simulink model "Vector_Control_SVPWM_encoderless_learn_v1_0"  (Simulink 10.0)
settings: Solver=ode23tb  StartTime=0.0  StopTime=2  FixedStep=Ts  RelTol=1e-3
PreLoadFcn:
  | %MotorParamInit_IM.m;
InitFcn:
  | Ts=1e-6;
  | %resolute=100;
  | 
  | run('MotorParamInit_IM.m');
undefined symbols (not defined in the file or in its folder): fN, J, Llr, Lls, np, PN, Rr, Rs, VN
libraries: powerlib x15, sfundemos x2, simulink x2, powerlib_extras x1
Description:
  | Copyright 2011-2013 Ruan Jiayang, Tsinghua Univ.
settings Model: Creator=Hoang Lehuy, Laval University  LastModifiedBy=W002220B  ExtModeTrigMode=oneshot  ExtModeArmWhenConnect=off  ExtModeAutoUpdateStatusClock=off
settings SolverCC: ZeroCrossControl=DisableAll
settings DataIOCC: SaveFinalState=on  SignalLoggingSaveFormat=ModelDataLogs  SaveOutput=off  SaveTime=off  SignalLoggingName=sigsOut
settings OptimizationCC: BlockReduction=off  ExpressionDepthLimit=2147483647  InitFltsAndDblsToZero=on
settings DebuggingCC: SaveWithParameterizedLinksMsg=none  CheckExecutionContextPreStartOutputMsg=on  CheckExecutionContextRuntimeOutputMsg=on  SignalResolutionControl=TryResolveAllWithWarning  MultiTaskDSMMsg=warning  MultiTaskCondExecSysMsg=none  FcnCallInpInsideContextMsg=warning  UnconnectedOutputMsg=none  StateNameClashWarn=warning
settings HardwareCC: TargetUnknown=on
settings SFSimCC: SimParseCustomCode=off
settings GRTTargetCC: TargetFcnLib=ansi_tfl_tmw.mat  GeneratePreprocessorConditionals=Disable all
settings ConfigComp: CovExternalEMLEnable=off
settings SimscapeCC: SimscapeNormalizeSystem=off

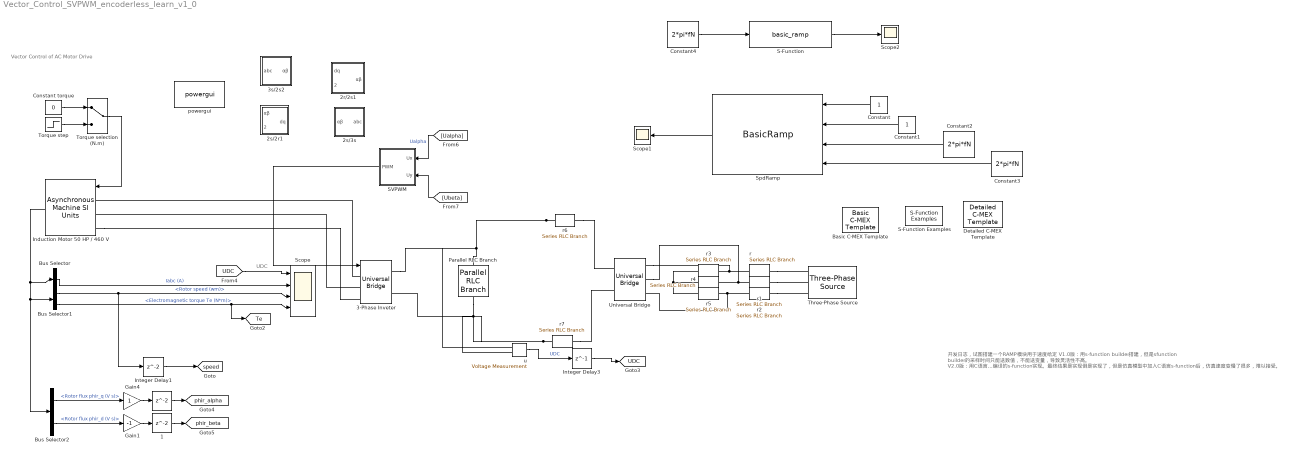
== system Vector_Control_SVPWM_encoderless_learn_v1_0 ==
  note: 开发日志，试图搭建一个RAMP模块用于速度给定
      | V1.0版：用s-function builder搭建，但是sfunction builder的采样时间只能送数值，不能送变量，导致灵活性不高。
      | V2.0版：用C语言编译的s-function实现。最终结果是实现倒是实现了，但是仿真模型中加入C语言s-function后，仿真速度变慢了很多，难以接受。
  note: Vector Control of AC Motor Drive
  note: UDC
  " " : Delay  InitialCondition=0  SampleTime=Ts
  " 1" : Delay  InitialCondition=0  SampleTime=Ts
  2r/2s1 : Subsystem
  2s/2r1 : Subsystem
  2s/3s : Subsystem
  3-Phase Inveter : powerlib/Power Electronics/Universal Bridge  Arms=3  SnubberResistance=1e5  SnubberCapacitance=1e-6  Device=IGBT / Diodes  Ron=1e-3  Lon=0  ForwardVoltages="[1.1  0.75]"  ForwardVoltage=0  GTOparameters=[ 10e-6 , 20e-6 ]  IGBTparameters=[ 1e-6 , 2e-6 ]  Measurements=None  Measurements_2=None  converterType=Rectifier
      settings: SourceProductName=Simscape Electrical
  3s/2s2 : Subsystem
  "Basic C-MEX Template " : sfundemos/C-file S-functions/Basic C-MEX Template   a=[]
  Bus Selector : BusSelector  OutputSignals=Stator measurements.Stator current is_a (A),Stator measurements.Stator current is_b (A),Stator measurements.Stator current is_c (A)  OutputAsBus=on
  Bus Selector1 : BusSelector  OutputSignals=Mechanical.Rotor speed (wm),Mechanical.Electromagnetic torque Te (N*m)
  Bus Selector2 : BusSelector  OutputSignals=Rotor measurements.Rotor flux phir_q (V s),Rotor measurements.Rotor flux phir_d (V s)
  Constant : Constant  SampleTime=Ts
  Constant torque : Constant  Value=0  SampleTime=Ts
  Constant1 : Constant
  Constant2 : Constant  Value=2*pi*fN
  Constant3 : Constant  Value=2*pi*fN
  Constant4 : Constant  Value=2*pi*fN
  Detailed C-MEX Template : sfundemos/C-file S-functions/Detailed C-MEX Template  a=[]
  Gain1 : Gain  Gain=-1
  Gain4 : Gain
  Induction Motor 50 HP / 460 V : powerlib/Machines/Asynchronous Machine SI Units  RotorType=Squirrel-cage  PresetModel=No  MechanicalLoad=Torque Tm  ShowDetailedParameters=on  ReferenceFrame=Rotor  Units=SI  MeasurementBus=off  NominalParameters=[PN, VN, fN]  Stator=[Rs Lls]  Rotor=[Rr Llr]  Cage1=[ 0.022 0.226/377]  Cage2=[ 0.022 0.226/377]  Lm=Lm  Mechanical=[J 0 np]  PolePairs=2  InitialConditions="[0, 0 ,  0 , 0 , 0 , 0 , 0 , 0 ]"  SimulateSaturation=off  Saturation=[0.6883 0.9028 1.1135 1.2559 1.3970 1.7538 2.1504 2.4988 2.6956 3.0579 3.7375 4.2552 5.1653 5.8110 6.5024;74.1928 98.0992 121.6600 137.3550 152.7109 190.0931 228.8721 259.2975 274.7375 301.8574 342.5384 366.6332 399.5942 417.9914 434.8974]  LoadFlowParameters=0  TsPowergui=0  TsBlock=Ts  IterativeModel=Forward Euler  IterativeDiscreteModel=Trapezoidal non iterative  Pmec=0
      settings: SourceProductName=Simscape Electrical
  Integer Delay1 : Delay  InitialCondition=0  SampleTime=Ts
  Integer Delay3 : Delay  DelayLength=1  InitialCondition=0  SampleTime=Ts
  Parallel RLC Branch : powerlib/Elements/Parallel RLC Branch  LConnTagsString=a  RConnTagsString=__new0  BranchType=RC  Resistance=330e3  Inductance=1e-3  SetiL0=off  InitialCurrent=0  Capacitance=330e-6*5  Setx0=on  InitialVoltage=530  Measurements=None
      settings: SourceProductName=Simscape Electrical
  S-Function : S-Function  FunctionName=basic_ramp  Parameters=Tup Tdown NormalValue Tsample  SFunctionDeploymentMode=off  EnableBusSupport=off  mask{Tup=1, Tdown=1, NormalValue=2*pi*fN, Tsample=1e-6}
      mask prompts: Tup "Ramp Up Time"; Tdown "Ramp Down Time"; NormalValue "Ramp Nominal Value"; Tsample "Ramp Module Excution Period"
  S-Function Examples : simulink/User-Defined Functions/S-Function Examples
      settings: SourceProductName=Simulink  SourceProductBaseCode=SL
  SVPWM : Subsystem  mask{DT=2e-6}
      mask prompts: DT "Dead Time (s)"
  Scope : Scope  NumInputPorts=4
  Scope1 : Scope
  Scope2 : Scope
  SpdRamp : S-Function  InitFcn=try, set_param(gcb,'FunctionName','BasicRamp'), end  FunctionName=BasicRamp  SFunctionModules=BasicRamp_wrapper  WizardData=DataTag0  SFunctionDeploymentMode=off  EnableBusSupport=off  mask(S-Function Builder){}
      mask help: Simulink:masks:SFunctionBuilder_MD
      mask init:
      | val = [[.9  0.75 0.75 1 1 .9 .9 1]',[1 1 0.75 0.75 .9 .9 1 .9]'];try , sys = get_param(gcb,'SfunBuilderFcnName');if isempty(sys), sys = get_param(gcb,'FunctionName'); end,catch, sys = get_param(gcb,'FunctionName'); end
      settings: CopyFcn=set_param(gcbh,'LinkStatus','none')  PreSaveFcn=try, set_param(gcb,'FunctionName','BasicRamp'), end  OpenFcn=sfunctionwizard(gcbh)
      mask Display: plot(val(:,1),val(:,2)),disp(sys), port_label('input',1,'RiseTime'), port_label('input',2,'FallTime'), port_label('input',3,'NormalValue'), port_label('input',4,'DestValue'), port_label('output',1,'RampOut')
  Three-Phase Source : powerlib/Electrical Sources/Three-Phase Source  InternalConnection=Yg  VoltagePhases=off  Voltage=380  PhaseAngle=0  Voltage_phases=[25e3 25e3 25e3]/sqrt(3)  PhaseAngles_phases=[0 -120 +120]  Frequency=50  NonIdealSource=on  SpecifyImpedance=off  Resistance=1e-5  Inductance=1e-6  ShortCircuitLevel=1e8  BaseVoltage=380  XRratio=0.1  BusType=swing  Pref=0  Qref=0  Prefabc=[10e3, 10e3, 10e3]  Qrefabc=[0, 0, 0]  Qmin=-inf  Qmax=inf
      settings: SourceProductName=Simscape Electrical
  Torque selection (N.m) : ManualSwitch
  Torque step : Step  After=5  SampleTime=Ts
  Universal Bridge : powerlib/Power Electronics/Universal Bridge  Arms=3  SnubberResistance=1e5  SnubberCapacitance=1e-6  Device=Diodes  Ron=1e-3  Lon=20e-9  ForwardVoltages="[  0  0  ]"  ForwardVoltage=0.7  GTOparameters=[ 10e-6 , 20e-6 ]  IGBTparameters=[ 1e-6 , 2e-6 ]  Measurements=None  Measurements_2=None  converterType=Rectifier
      settings: SourceProductName=Simscape Electrical
  powergui : powerlib/powergui  Priority=2  SimulationMode=Discrete  SampleTime=Ts  frequency=60  Iterations=50  frequencyindice=0  Pbase=100e6  ErrMax=1e-4  UnitsV=kV  UnitsW=MW  buscounter=0  FunctionMessages=off  echomessages=off  EnableUseOfTLC=off  CurrentSourceSwitches=off  DisableSnubberDevices=off  DisableRonSwitches=off  DisableVfSwitches=off  DisplayEquations=off  AutomaticDiscreteSolvers=off  SolverType=Tustin  Interpol=off  ExternalGateDelay=off  methode=off  Ts=0  x0status=blocks  SPID=off  SwTol=0  HookPort=off  NonlinearTolerance=1e-4  nMaxIteration=100  ContinueOnMaxIteration=off  RestoreLinks=warning  ResistiveCurrentMeasurement=off  Frange=[0:2:500]  Ylog=off  Xlog=off  ShowGrid=off  save=off  variable=ZData  structure=0  ZoomFFT=on  StartTime=0.0  cycles=1  DisplayStyle=off  fundamental=60  FreqAxis=off  MaxFrequency=1000  frequencyindicesteady=1  RmsSteady=1  display=off
      settings: SourceProductName=Simscape Electrical
  r : powerlib/Elements/Series RLC Branch  LConnTagsString=__new0  RConnTagsString=__new0  BranchType=L  Resistance=8e-6  Inductance=0.1e-3  SetiL0=off  InitialCurrent=0  Capacitance=1e-6  Setx0=off  InitialVoltage=0  Measurements=None
      settings: SourceProductName=Simscape Electrical
  r1 : powerlib/Elements/Series RLC Branch  LConnTagsString=__new0  RConnTagsString=__new0  BranchType=L  Resistance=8e-6  Inductance=0.1e-3  SetiL0=off  InitialCurrent=0  Capacitance=1e-6  Setx0=off  InitialVoltage=0  Measurements=None
      settings: SourceProductName=Simscape Electrical
  r2 : powerlib/Elements/Series RLC Branch  LConnTagsString=__new0  RConnTagsString=__new0  BranchType=L  Resistance=8e-6  Inductance=0.1e-3  SetiL0=off  InitialCurrent=0  Capacitance=1e-6  Setx0=off  InitialVoltage=0  Measurements=None
      settings: SourceProductName=Simscape Electrical
  r3 : powerlib/Elements/Series RLC Branch  LConnTagsString=__new0  RConnTagsString=__new0  BranchType=RC  Resistance=0.01  Inductance=1e-3  SetiL0=off  InitialCurrent=0  Capacitance=1e-6  Setx0=off  InitialVoltage=0  Measurements=None
      settings: SourceProductName=Simscape Electrical
  r4 : powerlib/Elements/Series RLC Branch  LConnTagsString=__new0  RConnTagsString=__new0  BranchType=RC  Resistance=0.01  Inductance=1e-3  SetiL0=off  InitialCurrent=0  Capacitance=1e-6  Setx0=off  InitialVoltage=0  Measurements=None
      settings: SourceProductName=Simscape Electrical
  r5 : powerlib/Elements/Series RLC Branch  LConnTagsString=__new0  RConnTagsString=__new0  BranchType=RC  Resistance=0.01  Inductance=1e-3  SetiL0=off  InitialCurrent=0  Capacitance=1e-6  Setx0=off  InitialVoltage=0  Measurements=None
      settings: SourceProductName=Simscape Electrical
  r6 : powerlib/Elements/Series RLC Branch  LConnTagsString=__new0  RConnTagsString=__new0  BranchType=RL  Resistance=1e-4  Inductance=1e-6  SetiL0=off  InitialCurrent=0  Capacitance=1e-6  Setx0=off  InitialVoltage=0  Measurements=None
      settings: SourceProductName=Simscape Electrical
  r7 : powerlib/Elements/Series RLC Branch  LConnTagsString=__new0  RConnTagsString=__new0  BranchType=RL  Resistance=1e-4  Inductance=1e-6  SetiL0=off  InitialCurrent=0  Capacitance=1e-6  Setx0=off  InitialVoltage=0  Measurements=None
      settings: SourceProductName=Simscape Electrical
  u : powerlib/Measurements/Voltage Measurement  Tag=PoWeRsYsTeMmEaSuReMeNt  PhasorSimulation=off  OutputType=Magnitude  PSBequivalent=0
      settings: SourceProductName=Simscape Electrical
  tag scope: Te=global, UDC=global, phir_alpha=global, phir_beta=global, speed=global
  wires:
  Bus Selector1/1 -> Scope/3, Integer Delay1/1  "<Rotor speed (wm)>"
  Torque step/1 -> Torque selection (N.m)/2
  Constant torque/1 -> Torque selection (N.m)/1
  Bus Selector/1 -> Scope/2  "Iabc (A)"
  Bus Selector1/2 -> Scope/4, [Te]  "<Electromagnetic torque Te (N*m)>"
  Torque selection (N.m)/1 -> Induction Motor 50 HP / 460 V/1
  Induction Motor 50 HP / 460 V/1 -> Bus Selector/1, Bus Selector1/1, Bus Selector2/1
  Integer Delay1/1 -> [speed]
  u/1 -> Integer Delay3/1  "UDC"
  SVPWM/1(PWM) -> 3-Phase Inveter/1
  [UDC] -> Scope/1
  Integer Delay3/1 -> [UDC]
  Bus Selector2/1 -> Gain4/1  "<Rotor flux phir_q (V s)>"
  Bus Selector2/2 -> Gain1/1  "<Rotor flux phir_d (V s)>"
  Gain4/1 -> " "/1
  " "/1 -> [phir_alpha]
  Gain1/1 -> " 1"/1
  " 1"/1 -> [phir_beta]
  [Ubeta] -> SVPWM/2(Uy)
  [Ualpha] -> SVPWM/1(Ux)  "Ualpha"
  Constant/1 -> SpdRamp/1
  Constant1/1 -> SpdRamp/2
  Constant2/1 -> SpdRamp/3
  Constant3/1 -> SpdRamp/4
  SpdRamp/1 -> Scope1/1
  S-Function/1 -> Scope2/1
  Constant4/1 -> S-Function/1
  connections:
  3-Phase Inveter/LConn1 -- Induction Motor 50 HP / 460 V/LConn1
  3-Phase Inveter/LConn2 -- Induction Motor 50 HP / 460 V/LConn2
  r6/LConn1 -- u/LConn1 -- 3-Phase Inveter/RConn1 -- Parallel RLC Branch/LConn1
  r7/LConn1 -- Parallel RLC Branch/RConn1 -- 3-Phase Inveter/RConn2 -- u/LConn2
  Universal Bridge/LConn1 -- r/LConn1 -- r3/RConn1
  r5/RConn1 -- Universal Bridge/LConn3 -- r2/LConn1
  Universal Bridge/LConn2 -- r1/LConn1 -- r4/RConn1
  r/RConn1 -- Three-Phase Source/RConn1
  r1/RConn1 -- Three-Phase Source/RConn2
  r3/LConn1 -- r4/LConn1 -- r5/LConn1
  r2/RConn1 -- Three-Phase Source/RConn3
  r6/RConn1 -- Universal Bridge/RConn1
  r7/RConn1 -- Universal Bridge/RConn2
  Induction Motor 50 HP / 460 V/LConn3 -- 3-Phase Inveter/LConn3

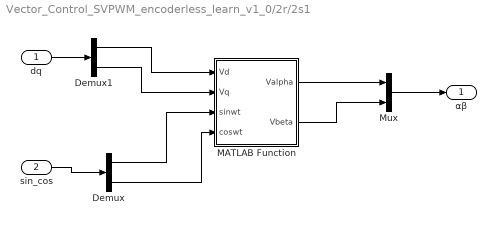
== system Vector_Control_SVPWM_encoderless_learn_v1_0/2r/2s1 ==
  dq : Inport
  sin_cos : Inport  Port=2
  Demux : Demux  Outputs=2
  Demux1 : Demux  Outputs=2
  MATLAB Function : MATLAB Function  TreatAsAtomicUnit=on
  Mux : Mux  Inputs=2
  αβ : Outport
  wires:
  MATLAB Function/2(Vbeta) -> Mux/2
  MATLAB Function/1(Valpha) -> Mux/1
  Demux1/2 -> MATLAB Function/2(Vq)
  Demux1/1 -> MATLAB Function/1(Vd)
  dq/1 -> Demux1/1
  sin_cos/1 -> Demux/1
  Demux/1 -> MATLAB Function/3(sinwt)
  Demux/2 -> MATLAB Function/4(coswt)
  Mux/1 -> αβ/1

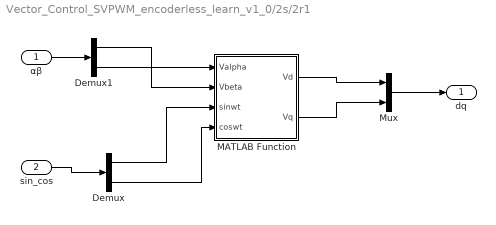
== system Vector_Control_SVPWM_encoderless_learn_v1_0/2s/2r1 ==
  αβ : Inport
  sin_cos : Inport  Port=2
  Demux : Demux  Outputs=2
  Demux1 : Demux  Outputs=2
  MATLAB Function : MATLAB Function  TreatAsAtomicUnit=on
  Mux : Mux  Inputs=2
  dq : Outport
  wires:
  Demux1/1 -> MATLAB Function/1(Valpha)
  Demux1/2 -> MATLAB Function/2(Vbeta)
  Mux/1 -> dq/1
  MATLAB Function/2(Vq) -> Mux/2
  MATLAB Function/1(Vd) -> Mux/1
  Demux/2 -> MATLAB Function/4(coswt)
  Demux/1 -> MATLAB Function/3(sinwt)
  sin_cos/1 -> Demux/1
  αβ/1 -> Demux1/1

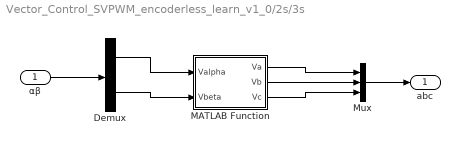
== system Vector_Control_SVPWM_encoderless_learn_v1_0/2s/3s ==
  αβ : Inport
  Demux : Demux  Outputs=2
  MATLAB Function : MATLAB Function  TreatAsAtomicUnit=on
  Mux : Mux  Inputs=3
  abc : Outport
  wires:
  Demux/1 -> MATLAB Function/1(Valpha)
  Demux/2 -> MATLAB Function/2(Vbeta)
  MATLAB Function/1(Va) -> Mux/1
  MATLAB Function/2(Vb) -> Mux/2
  MATLAB Function/3(Vc) -> Mux/3
  Mux/1 -> abc/1
  αβ/1 -> Demux/1

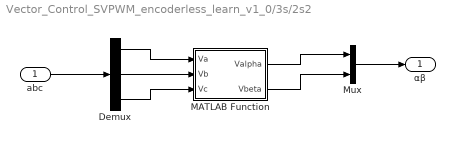
== system Vector_Control_SVPWM_encoderless_learn_v1_0/3s/2s2 ==
  abc : Inport
  Demux : Demux  Outputs=3
  MATLAB Function : MATLAB Function  TreatAsAtomicUnit=on
  Mux : Mux  Inputs=2
  αβ : Outport
  wires:
  abc/1 -> Demux/1
  Mux/1 -> αβ/1
  Demux/1 -> MATLAB Function/1(Va)
  Demux/2 -> MATLAB Function/2(Vb)
  Demux/3 -> MATLAB Function/3(Vc)
  MATLAB Function/1(Valpha) -> Mux/1
  MATLAB Function/2(Vbeta) -> Mux/2

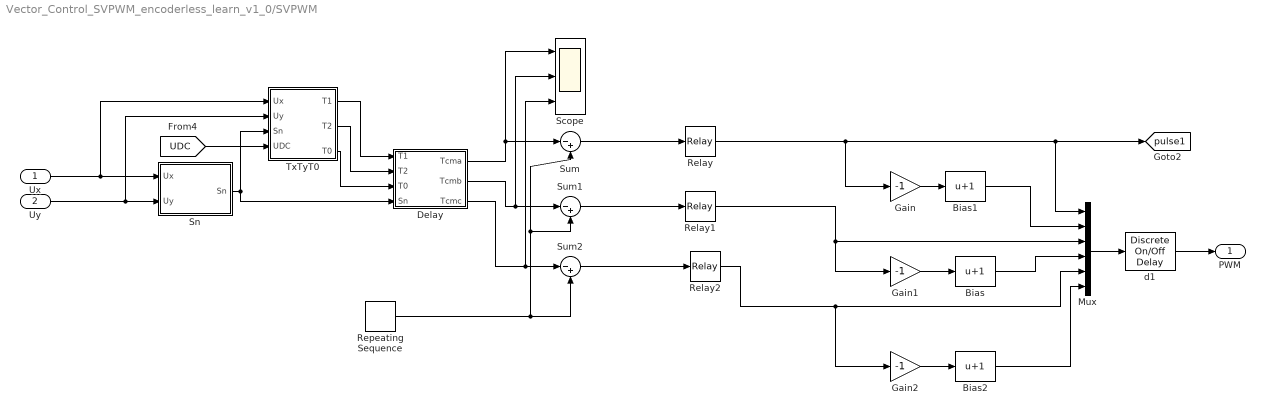
== system Vector_Control_SVPWM_encoderless_learn_v1_0/SVPWM ==
  Ux : Inport
  Uy : Inport  Port=2
  Bias : Bias  Bias=1
  Bias1 : Bias  Bias=1
  Bias2 : Bias  Bias=1
  Delay : MATLAB Function  TreatAsAtomicUnit=on
  Gain : Gain  Gain=-1
  Gain1 : Gain  Gain=-1
  Gain2 : Gain  Gain=-1
  Mux : Mux  Inputs=6
  Relay : Relay  OnSwitchValue=0  OffSwitchValue=0
  Relay1 : Relay  OnSwitchValue=0  OffSwitchValue=0
  Relay2 : Relay  OnSwitchValue=0  OffSwitchValue=0
  Repeating Sequence : simulink/Sources/Repeating Sequence  rep_seq_t=[0 1/5000/2 1/5000]  rep_seq_y=[0 1/5000/2 0]
  Scope : Scope  NumInputPorts=3
  Sn : MATLAB Function  TreatAsAtomicUnit=on
  Sum : Sum  Inputs=|-+
  Sum1 : Sum  Inputs=|-+
  Sum2 : Sum  Inputs=|-+
  TxTyT0 : MATLAB Function  TreatAsAtomicUnit=on
  d1 : powerlib_extras/Discrete  Control Blocks/Discrete On//Off Delay  type_delay=On delay  delay=DT  ic=0  Ts=Ts
      settings: SourceProductName=Simscape Electrical  SourceProductBaseCode=PS
  PWM : Outport
  tag scope: pulse1=global
  wires:
  Delay/1(Tcma) -> Sum/1, Scope/1
  Delay/2(Tcmb) -> Sum1/1, Scope/2
  Delay/3(Tcmc) -> Sum2/1, Scope/3
  Repeating Sequence/1 -> Sum/2, Sum1/2, Sum2/2
  Sum/1 -> Relay/1
  Sum2/1 -> Relay2/1
  Sum1/1 -> Relay1/1
  Relay1/1 -> Gain1/1, Mux/3
  Relay2/1 -> Gain2/1, Mux/5
  Sn/1(Sn) -> TxTyT0/3(Sn), Delay/4(Sn)
  TxTyT0/1(T1) -> Delay/1(T1)
  TxTyT0/2(T2) -> Delay/2(T2)
  TxTyT0/3(T0) -> Delay/3(T0)
  Gain1/1 -> Bias/1
  Gain/1 -> Bias1/1
  Gain2/1 -> Bias2/1
  Relay/1 -> Gain/1, Mux/1, [pulse1]
  Ux/1 -> Sn/1(Ux), TxTyT0/1(Ux)
  Uy/1 -> Sn/2(Uy), TxTyT0/2(Uy)
  [UDC] -> TxTyT0/4(UDC)
  Bias1/1 -> Mux/2
  Bias/1 -> Mux/4
  Bias2/1 -> Mux/6
  d1/1 -> PWM/1
  Mux/1 -> d1/1

== matlab function SVPWM/Sn ==
  data: Sn output double; Ux input double; Uy input double
function Sn = S(Ux,Uy)
theta=atan2(Uy,Ux)*180/pi;
if theta>=0&&theta<60
    Sn=1;
elseif theta>=60&&theta<120
    Sn=2;
elseif theta>=120&&theta<180
    Sn=3;
elseif theta>=-180&&theta<-120
    Sn=4;
elseif theta>=-120&&theta<-60
    Sn=5;
else Sn=6;
end

== matlab function SVPWM/TxTyT0 ==
  data: Ux input double; Uy input double; Sn input double; T1 output double; T2 output double; T0 output double; UDC input double
function [T1,T2,T0]=T(Ux,Uy,Sn,UDC)
Ts=1/5000;
Udc=UDC;

X=sqrt(3)*Ts/Udc*Uy;
Y=sqrt(3)*Ts/2/Udc*(sqrt(3)*Ux+Uy);
Z=sqrt(3)*Ts/2/Udc*(-sqrt(3)*Ux+Uy);

if Sn==1
    T1=-Z;T2=X;
elseif Sn==2;
    T1=Z;T2=Y;
elseif Sn==3;
    T1=X;T2=-Y;
elseif Sn==4;
    T1=-X;T2=Z;
elseif Sn==5;
    T1=-Y;T2=-Z;
else T1=Y;T2=-X;
end
    
if T1+T2>Ts
    a=T1;b=T2;
    T1=a*Ts/(a+b);
    T2=b*Ts/(a+b);
end

T0=Ts-T1-T2;

== matlab function SVPWM/Delay ==
  data: T1 input double; T2 input double; T0 input double; Tcma output double; Tcmb output double; Tcmc output double; Sn input double
function [Tcma,Tcmb,Tcmc]=D(T1,T2,T0,Sn)
T=1/5000;
ton1=0.25*T0;
ton2=ton1+T1/2;
ton3=ton2+T2/2;
if Sn==1
    Tcma=ton1;Tcmb=ton2;Tcmc=ton3;
elseif Sn==2;
    Tcma=ton2;Tcmb=ton1;Tcmc=ton3;
elseif Sn==3;
    Tcma=ton3;Tcmb=ton1;Tcmc=ton2;
elseif Sn==4;
    Tcma=ton3;Tcmb=ton2;Tcmc=ton1;
elseif Sn==5;
    Tcma=ton2;Tcmb=ton3;Tcmc=ton1;
else Tcma=ton1;Tcmb=ton3;Tcmc=ton2;
end

== matlab function 2s//3s/MATLAB Function ==
  data: Va output double; Valpha input double; Vb output double; Vc output double; Vbeta input double
function [Va, Vb, Vc] = Park(Valpha, Vbeta)
%#codegen
Va = sqrt(2/3)*Valpha;
Vb = -Valpha/sqrt(6) + Vbeta/sqrt(2);
Vc = -Valpha/sqrt(6) - Vbeta/sqrt(2);

== matlab function 3s//2s2/MATLAB Function ==
  data: Va input double; Valpha output double; Vb input double; Vc input double; Vbeta output double
function [Valpha, Vbeta] = Park(Va, Vb, Vc)
%#codegen
Valpha = sqrt(2/3)*(Va - Vb/2 -Vc/2);
Vbeta  = sqrt(2/3)*(sqrt(3)*Vb/2 - sqrt(3)*Vc/2);

== matlab function 2r//2s1/MATLAB Function ==
  data: Valpha output double; Vd input double; Vbeta output double; Vq input double; sinwt input double; coswt input double
function [Valpha, Vbeta] = fcn(Vd, Vq, sinwt, coswt)
%#codegen

Valpha = Vd*coswt - Vq*sinwt;
Vbeta  = Vd*sinwt + Vq*coswt;

== matlab function 2s//2r1/MATLAB Function ==
  data: Valpha input double; Vd output double; Vbeta input double; Vq output double; sinwt input double; coswt input double
function [Vd, Vq] = fcn(Valpha, Vbeta, sinwt, coswt)
%#codegen

Vd =  Valpha*coswt + Vbeta*sinwt;
Vq = -Valpha*sinwt + Vbeta*coswt;
